simulink model "SRRF"  (R2013a)
settings: Solver=ode4  StartTime=0.0  StopTime=2  FixedStep=1/25600  RelTol=1e-3
libraries: powerlib_meascontrol x27, simulink x8, powerlib x1
settings Model: Creator=Eren  LastModifiedBy=erencan

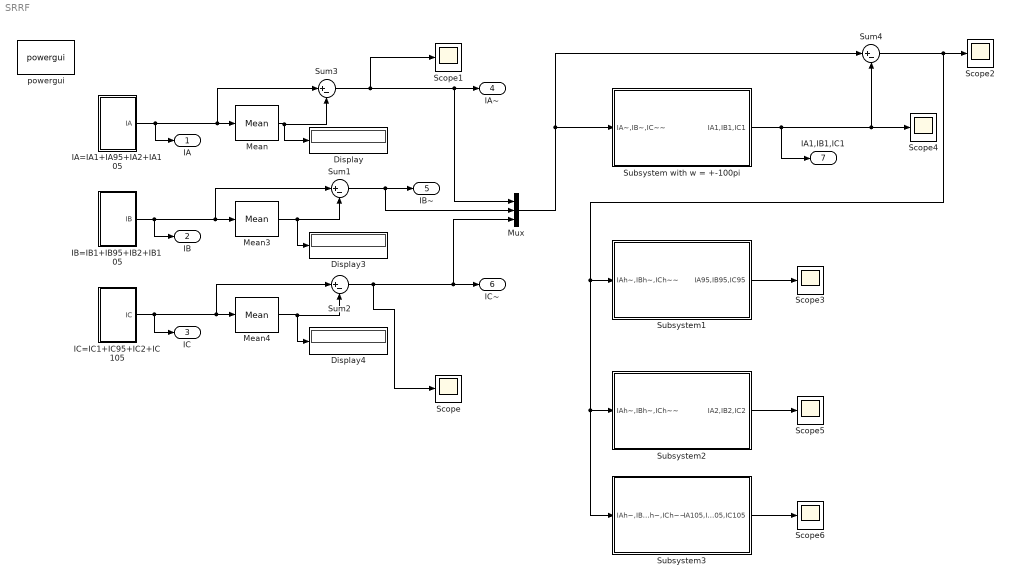
== system SRRF ==
  Display : Display
  Display3 : Display
  Display4 : Display
  "IA=IA1+IA95+IA2+IA105 " : Subsystem
  "IB=IB1+IB95+IB2+IB105 " : Subsystem
  "IC=IC1+IC95+IC2+IC105 " : Subsystem
  Mean : powerlib_meascontrol/Measurements/Mean  Freq=50  Vinit=0  Ts=0
  Mean3 : powerlib_meascontrol/Measurements/Mean  Freq=50  Vinit=0  Ts=0
  Mean4 : powerlib_meascontrol/Measurements/Mean  Freq=50  Vinit=0  Ts=0
  Mux : Mux  Inputs=3
  Scope{,1..6} (7 alike) : Scope
      Scope settings: YMin=-3000  YMax=3000
      Scope2 settings: YMin=-3000  YMax=3000  SaveName=ScopeData5
      Scope3 settings: YMin=-3000  YMax=3000  SaveName=ScopeData6
      Scope4 settings: YMin=-3000  YMax=3000  SaveName=ScopeData7
      Scope5 settings: YMin=-3000  YMax=3000  SaveName=ScopeData8
      Scope6 settings: YMin=-3000  YMax=3000  SaveName=ScopeData9
  Subsystem with w = +-100pi : Subsystem
  Subsystem1 : Subsystem
  Subsystem2 : Subsystem
  Subsystem3 : Subsystem
  Sum{1..4} (4 alike) : Sum  Inputs=|+-
  powergui : powerlib/powergui  Priority=1  SimulationMode=Continuous  SolverType=Tustin  SampleTime=50e-6  frequency=60  SPID=off  DisableSnubberDevices=off  DisableRonSwitches=off  DisableVfSwitches=off  SwTol=0  Interpol=off  DisplayEquations=off  frequencyindice=50  Pbase=100e6  ErrMax=1e-4  Iterations=50  UnitsV=kV  UnitsW=MW  FunctionMessages=off  echomessages=off  HookPort=off  EnableUseOfTLC=off  x0status=blocks  RestoreLinks=warning  ResistiveCurrentMeasurement=off  Frange=[0:2:500]  Ylog=off  Xlog=on  ShowGrid=off  save=off  variable=ZData  ZoomFFT=off  StartTime=0.0  cycles=1  DisplayStyle=1  fundamental=60  FreqAxis=off  MaxFrequency=1000  frequencyindicesteady=1  RmsSteady=1  display=off  Ts=0  methode=off
  IA : Outport
  "IB " : Outport  Port=2
  "IC " : Outport  Port=3
  "IA~ " : Outport  Port=4
  IB~ : Outport  Port=5
  IC~ : Outport  Port=6
  IA1,IB1,IC1 : Outport  Port=7
  wires:
  Mean/1 -> Sum3/2, Display/1
  "IA=IA1+IA95+IA2+IA105 "/1(IA) -> Sum3/1, Mean/1, IA/1
  "IB=IB1+IB95+IB2+IB105 "/1("IB ") -> Sum1/1, Mean3/1, "IB "/1
  Sum3/1 -> Scope1/1, Mux/1, "IA~ "/1
  Mean3/1 -> Sum1/2, Display3/1
  Sum1/1 -> Mux/2, IB~/1
  "IC=IC1+IC95+IC2+IC105 "/1("IC ") -> Sum2/1, Mean4/1, "IC "/1
  Mean4/1 -> Sum2/2, Display4/1
  Sum2/1 -> Scope/1, Mux/3, IC~/1
  Mux/1 -> Sum4/1, Subsystem with w = +-100pi/1(IA~,IB~,IC~~)
  Subsystem with w = +-100pi/1(IA1,IB1,IC1) -> IA1,IB1,IC1/1, Sum4/2, Scope4/1
  Sum4/1 -> Subsystem1/1(IAh~,IBh~,ICh~~), Subsystem2/1(IAh~,IBh~,ICh~~), Subsystem3/1(IAh~,IBh~,ICh~~), Scope2/1
  Subsystem1/1("IA95,IB95,IC95 ") -> Scope3/1
  Subsystem2/1("IA2,IB2,IC2 ") -> Scope5/1
  Subsystem3/1("IA105,IB105,IC105 ") -> Scope6/1

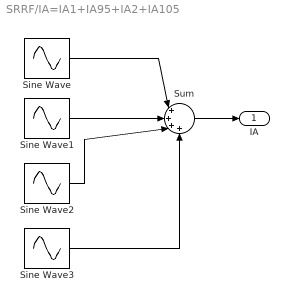
== system SRRF/IA=IA1+IA95+IA2+IA105  ==
  Sine Wave : Sin  Amplitude=1750*sqrt(2)  Frequency=100*pi  SampleTime=0  VectorParams1D=off
  Sine Wave1 : Sin  Amplitude=190*sqrt(2)  Frequency=190*pi  SampleTime=0  VectorParams1D=off
  Sine Wave2 : Sin  Amplitude=154*sqrt(2)  Frequency=200*pi  SampleTime=0  VectorParams1D=off
  Sine Wave3 : Sin  Amplitude=180*sqrt(2)  Frequency=210*pi  SampleTime=0  VectorParams1D=off
  Sum : Sum  Inputs=|++++
  IA : Outport
  wires:
  Sum/1 -> IA/1
  Sine Wave2/1 -> Sum/3
  Sine Wave/1 -> Sum/1
  Sine Wave3/1 -> Sum/4
  Sine Wave1/1 -> Sum/2

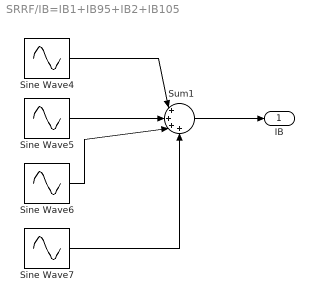
== system SRRF/IB=IB1+IB95+IB2+IB105  ==
  Sine Wave4 : Sin  Amplitude=1261.9*sqrt(2)  Frequency=100*pi  Phase=-0.7439*pi  SampleTime=0  VectorParams1D=off
  Sine Wave5 : Sin  Amplitude=95.4*sqrt(2)  Frequency=190*pi  Phase=-0.9711*pi  SampleTime=0  VectorParams1D=off
  Sine Wave6 : Sin  Amplitude=77.95*sqrt(2)  Frequency=200*pi  Phase=-0.9503*pi  SampleTime=0  VectorParams1D=off
  Sine Wave7 : Sin  Amplitude=96.4*sqrt(2)  Frequency=210*pi  Phase=-0.883*pi  SampleTime=0  VectorParams1D=off
  Sum1 : Sum  Inputs=|++++
  "IB " : Outport
  wires:
  Sum1/1 -> "IB "/1
  Sine Wave5/1 -> Sum1/2
  Sine Wave4/1 -> Sum1/1
  Sine Wave6/1 -> Sum1/3
  Sine Wave7/1 -> Sum1/4

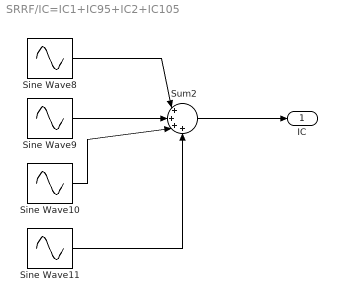
== system SRRF/IC=IC1+IC95+IC2+IC105  ==
  Sine Wave10 : Sin  Amplitude=77.95*sqrt(2)  Frequency=200*pi  Phase=0.9503*pi  SampleTime=0  VectorParams1D=off
  Sine Wave11 : Sin  Amplitude=96.4*sqrt(2)  Frequency=210*pi  Phase=0.883*pi  SampleTime=0  VectorParams1D=off
  Sine Wave8 : Sin  Amplitude=1261.9*sqrt(2)  Frequency=100*pi  Phase=0.7439*pi  SampleTime=0  VectorParams1D=off
  Sine Wave9 : Sin  Amplitude=95.4*sqrt(2)  Frequency=190*pi  Phase=0.9711*pi  SampleTime=0  VectorParams1D=off
  Sum2 : Sum  Inputs=|++++
  "IC " : Outport
  wires:
  Sine Wave11/1 -> Sum2/4
  Sine Wave10/1 -> Sum2/3
  Sine Wave9/1 -> Sum2/2
  Sine Wave8/1 -> Sum2/1
  Sum2/1 -> "IC "/1

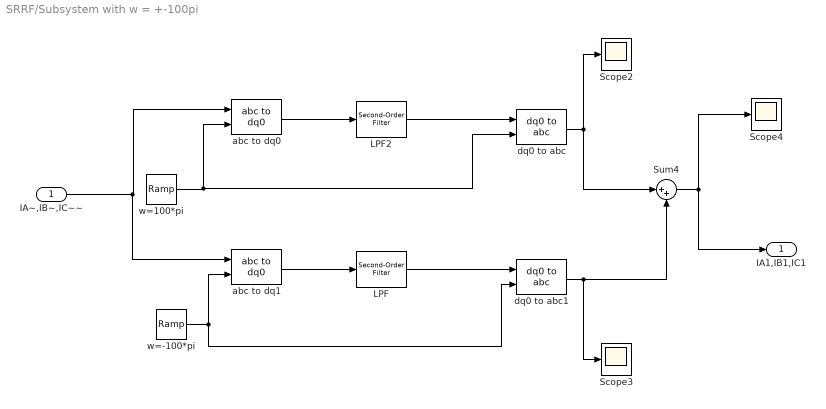
== system SRRF/Subsystem with w = +-100pi ==
  IA~,IB~,IC~~ : Inport
  LPF : powerlib_meascontrol/Filters/Second-Order Filter  FilterType=Lowpass  Fo=2.5  Zeta=0.707  Ts=0  Initialize=on  Vac_Init="[0,  0,  60]"  Vdc_Init=0  PlotResponse=off  FreqRange=[0, 500, 1]
  "LPF2 " : powerlib_meascontrol/Filters/Second-Order Filter  FilterType=Lowpass  Fo=2.5  Zeta=0.707  Ts=0  Initialize=on  Vac_Init="[0,  0,  60]"  Vdc_Init=0  PlotResponse=off  FreqRange=[0, 500, 1]
  Scope2 : Scope
      settings: YMin=-3000  YMax=3000  SaveName=ScopeData2
  Scope3 : Scope
      settings: YMin=-3000  YMax=3000  SaveName=ScopeData3
  Scope4 : Scope
      settings: YMin=-3000  YMax=3000  SaveName=ScopeData4
  Sum4 : Sum  Inputs=|++
  abc to dq0 : powerlib_meascontrol/Transformations/abc to dq0  Alignment=90 degrees behind phase A axis
  abc to dq1 : powerlib_meascontrol/Transformations/abc to dq0  Alignment=90 degrees behind phase A axis
  dq0 to abc : powerlib_meascontrol/Transformations/dq0 to abc  Alignment=90 degrees behind phase A axis
  dq0 to abc1 : powerlib_meascontrol/Transformations/dq0 to abc  Alignment=90 degrees behind phase A axis
  "w=-100*pi " : simulink/Sources/Ramp  slope=-100*pi  start=0  X0=0
  "w=100*pi " : simulink/Sources/Ramp  slope=100*pi  start=0  X0=0
  IA1,IB1,IC1 : Outport
  wires:
  Sum4/1 -> IA1,IB1,IC1/1, Scope4/1
  dq0 to abc1/1 -> Sum4/2, Scope3/1
  dq0 to abc/1 -> Sum4/1, Scope2/1
  abc to dq1/1 -> LPF/1
  abc to dq0/1 -> "LPF2 "/1
  "LPF2 "/1 -> dq0 to abc/1
  LPF/1 -> dq0 to abc1/1
  IA~,IB~,IC~~/1 -> abc to dq1/1, abc to dq0/1
  "w=100*pi "/1 -> dq0 to abc/2, abc to dq0/2
  "w=-100*pi "/1 -> abc to dq1/2, dq0 to abc1/2

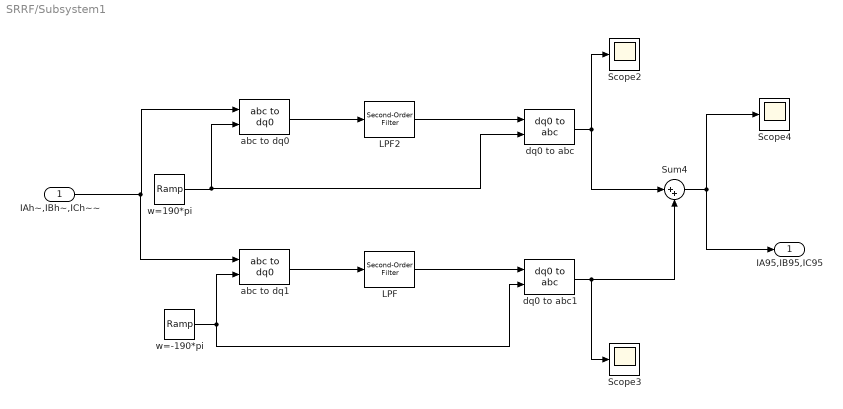
== system SRRF/Subsystem1 ==
  IAh~,IBh~,ICh~~ : Inport
  LPF : powerlib_meascontrol/Filters/Second-Order Filter  FilterType=Lowpass  Fo=2.5  Zeta=0.707  Ts=0  Initialize=on  Vac_Init="[0,  0,  60]"  Vdc_Init=0  PlotResponse=off  FreqRange=[0, 500, 1]
  "LPF2 " : powerlib_meascontrol/Filters/Second-Order Filter  FilterType=Lowpass  Fo=2.5  Zeta=0.707  Ts=0  Initialize=on  Vac_Init="[0,  0,  60]"  Vdc_Init=0  PlotResponse=off  FreqRange=[0, 500, 1]
  Scope2 : Scope
      settings: YMin=-3000  YMax=3000  SaveName=ScopeData2
  Scope3 : Scope
      settings: YMin=-3000  YMax=3000  SaveName=ScopeData3
  Scope4 : Scope
      settings: YMin=-3000  YMax=3000  SaveName=ScopeData4
  Sum4 : Sum  Inputs=|++
  abc to dq0 : powerlib_meascontrol/Transformations/abc to dq0  Alignment=90 degrees behind phase A axis
  abc to dq1 : powerlib_meascontrol/Transformations/abc to dq0  Alignment=90 degrees behind phase A axis
  dq0 to abc : powerlib_meascontrol/Transformations/dq0 to abc  Alignment=90 degrees behind phase A axis
  dq0 to abc1 : powerlib_meascontrol/Transformations/dq0 to abc  Alignment=90 degrees behind phase A axis
  "w=-190*pi " : simulink/Sources/Ramp  slope=-190*pi  start=0  X0=0
  "w=190*pi " : simulink/Sources/Ramp  slope=190*pi  start=0  X0=0
  "IA95,IB95,IC95 " : Outport
  wires:
  Sum4/1 -> "IA95,IB95,IC95 "/1, Scope4/1
  dq0 to abc1/1 -> Sum4/2, Scope3/1
  dq0 to abc/1 -> Sum4/1, Scope2/1
  abc to dq1/1 -> LPF/1
  abc to dq0/1 -> "LPF2 "/1
  "LPF2 "/1 -> dq0 to abc/1
  LPF/1 -> dq0 to abc1/1
  IAh~,IBh~,ICh~~/1 -> abc to dq1/1, abc to dq0/1
  "w=190*pi "/1 -> dq0 to abc/2, abc to dq0/2
  "w=-190*pi "/1 -> abc to dq1/2, dq0 to abc1/2

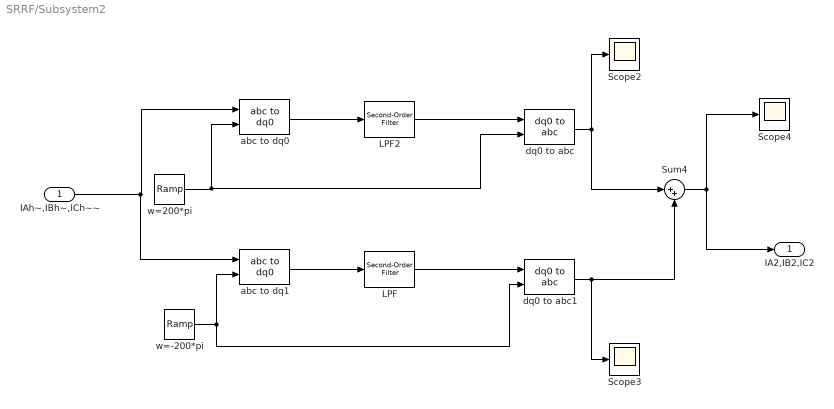
== system SRRF/Subsystem2 ==
  IAh~,IBh~,ICh~~ : Inport
  LPF : powerlib_meascontrol/Filters/Second-Order Filter  FilterType=Lowpass  Fo=2.5  Zeta=0.707  Ts=0  Initialize=on  Vac_Init="[0,  0,  60]"  Vdc_Init=0  PlotResponse=off  FreqRange=[0, 500, 1]
  "LPF2 " : powerlib_meascontrol/Filters/Second-Order Filter  FilterType=Lowpass  Fo=2.5  Zeta=0.707  Ts=0  Initialize=on  Vac_Init="[0,  0,  60]"  Vdc_Init=0  PlotResponse=off  FreqRange=[0, 500, 1]
  Scope2 : Scope
      settings: YMin=-3000  YMax=3000  SaveName=ScopeData2
  Scope3 : Scope
      settings: YMin=-3000  YMax=3000  SaveName=ScopeData3
  Scope4 : Scope
      settings: YMin=-3000  YMax=3000  SaveName=ScopeData4
  Sum4 : Sum  Inputs=|++
  abc to dq0 : powerlib_meascontrol/Transformations/abc to dq0  Alignment=90 degrees behind phase A axis
  abc to dq1 : powerlib_meascontrol/Transformations/abc to dq0  Alignment=90 degrees behind phase A axis
  dq0 to abc : powerlib_meascontrol/Transformations/dq0 to abc  Alignment=90 degrees behind phase A axis
  dq0 to abc1 : powerlib_meascontrol/Transformations/dq0 to abc  Alignment=90 degrees behind phase A axis
  "w=-200*pi " : simulink/Sources/Ramp  slope=-200*pi  start=0  X0=0
  "w=200*pi " : simulink/Sources/Ramp  slope=200*pi  start=0  X0=0
  "IA2,IB2,IC2 " : Outport
  wires:
  Sum4/1 -> "IA2,IB2,IC2 "/1, Scope4/1
  dq0 to abc1/1 -> Sum4/2, Scope3/1
  dq0 to abc/1 -> Sum4/1, Scope2/1
  abc to dq1/1 -> LPF/1
  abc to dq0/1 -> "LPF2 "/1
  "LPF2 "/1 -> dq0 to abc/1
  LPF/1 -> dq0 to abc1/1
  IAh~,IBh~,ICh~~/1 -> abc to dq1/1, abc to dq0/1
  "w=200*pi "/1 -> dq0 to abc/2, abc to dq0/2
  "w=-200*pi "/1 -> abc to dq1/2, dq0 to abc1/2

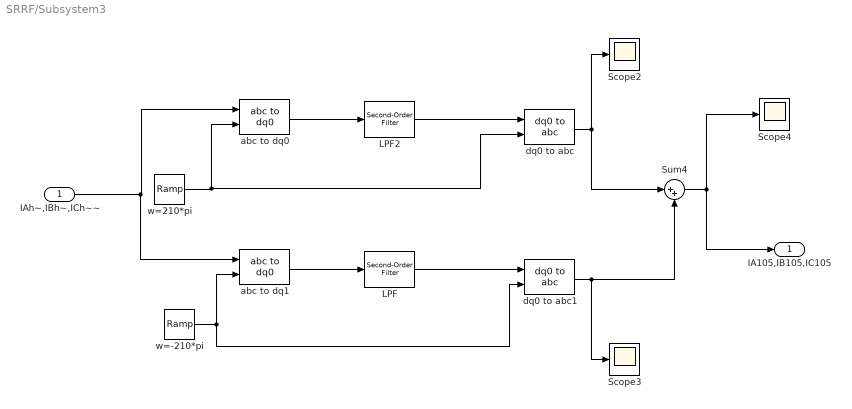
== system SRRF/Subsystem3 ==
  IAh~,IBh~,ICh~~ : Inport
  LPF : powerlib_meascontrol/Filters/Second-Order Filter  FilterType=Lowpass  Fo=2.5  Zeta=0.707  Ts=0  Initialize=on  Vac_Init="[0,  0,  60]"  Vdc_Init=0  PlotResponse=off  FreqRange=[0, 500, 1]
  "LPF2 " : powerlib_meascontrol/Filters/Second-Order Filter  FilterType=Lowpass  Fo=2.5  Zeta=0.707  Ts=0  Initialize=on  Vac_Init="[0,  0,  60]"  Vdc_Init=0  PlotResponse=off  FreqRange=[0, 500, 1]
  Scope2 : Scope
      settings: YMin=-3000  YMax=3000  SaveName=ScopeData2
  Scope3 : Scope
      settings: YMin=-3000  YMax=3000  SaveName=ScopeData3
  Scope4 : Scope
      settings: YMin=-3000  YMax=3000  SaveName=ScopeData4
  Sum4 : Sum  Inputs=|++
  abc to dq0 : powerlib_meascontrol/Transformations/abc to dq0  Alignment=90 degrees behind phase A axis
  abc to dq1 : powerlib_meascontrol/Transformations/abc to dq0  Alignment=90 degrees behind phase A axis
  dq0 to abc : powerlib_meascontrol/Transformations/dq0 to abc  Alignment=90 degrees behind phase A axis
  dq0 to abc1 : powerlib_meascontrol/Transformations/dq0 to abc  Alignment=90 degrees behind phase A axis
  "w=-210*pi " : simulink/Sources/Ramp  slope=-210*pi  start=0  X0=0
  "w=210*pi " : simulink/Sources/Ramp  slope=210*pi  start=0  X0=0
  "IA105,IB105,IC105 " : Outport
  wires:
  Sum4/1 -> "IA105,IB105,IC105 "/1, Scope4/1
  dq0 to abc1/1 -> Sum4/2, Scope3/1
  dq0 to abc/1 -> Sum4/1, Scope2/1
  abc to dq1/1 -> LPF/1
  abc to dq0/1 -> "LPF2 "/1
  "LPF2 "/1 -> dq0 to abc/1
  LPF/1 -> dq0 to abc1/1
  IAh~,IBh~,ICh~~/1 -> abc to dq1/1, abc to dq0/1
  "w=210*pi "/1 -> dq0 to abc/2, abc to dq0/2
  "w=-210*pi "/1 -> abc to dq1/2, dq0 to abc1/2
